simulink model "PV_MPPT"  (R2023a)
settings: Solver=VariableStepAuto  StartTime=0.0  StopTime=2  RelTol=1e-3
undefined symbols (not defined in the file): Ion, Lithium
libraries: spsSeriesRLCBranchLib x4, spsVariableResistorLib x2, spsVoltageMeasurementLib x2, spsBatteryLib x1, spsCurrentMeasurementLib x1, spsDiodeLib x1, spsIGBTLib x1, spsPVArrayLib x1, spspowerguiLib x1
settings Model: Creator=adity  LastModifiedBy=hp
settings RTWCC: GPUComputeCapability=5.0

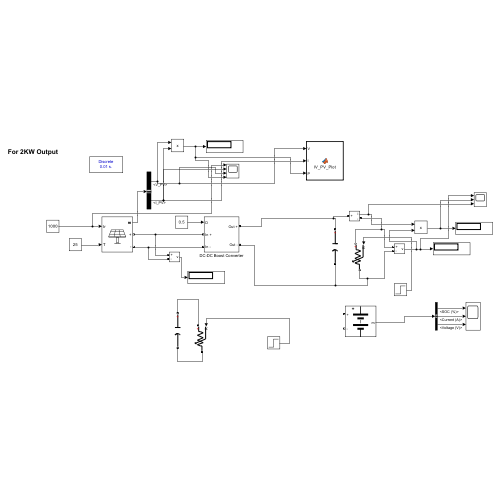
[thumbnail: Simulink's stored preview of the top-level diagram]
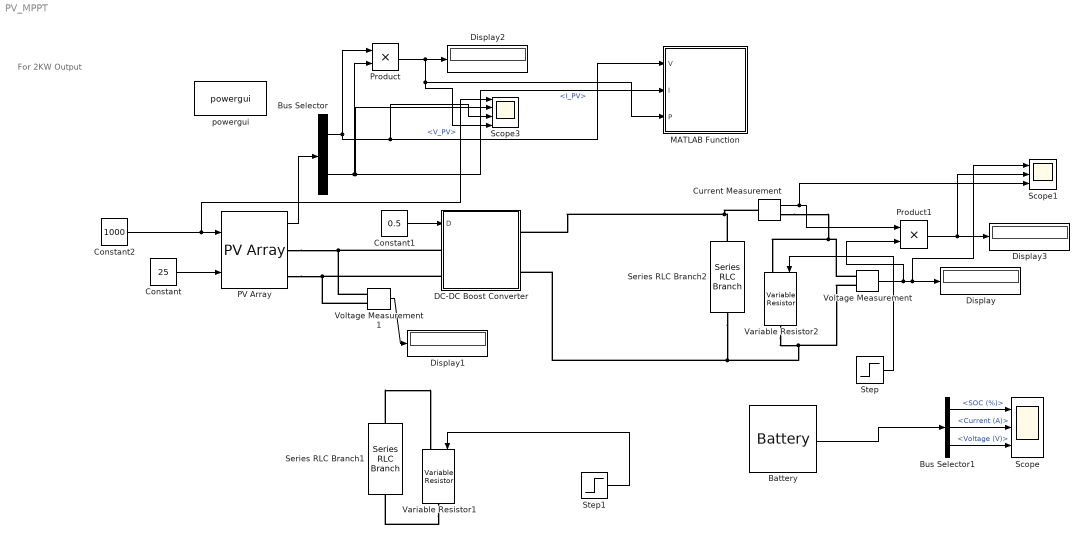
== system PV_MPPT ==
  note: For 2KW Output
  Battery : spsBatteryLib/Battery  BatType=Lithium-Ion  ShowTempParam=off  ThermalPreset=no  ShowAgeParam=off  NomV=7.2  NomQ=5.4  SOC=50  Batt_Tr=30  PresetModel=on  MaxQ=5.4  MinV=5.4  FullV=8.3807  Dis_rate=2.3478  R=0.013333  Normal_OP=4.8835  expZone="[7.7788      0.2653]"  current=[6.5 13 32.5]  Units=Time  Tci=20  NomT=20  T2=-30  MaxQ2=4.8  FullV2=7.1  Normal_OP2=5.655  expZone2="[6.58           1]"  Rca=0.6  ti=2000  Dp=0  Neq0=0  Tsim=1e6  Ta1=25  Qeol=5.4*0.9  Reol=0.013333*1.2  Char_age=[2.3478, 3]  Dis_age=[2.3478, 10]  N1=1500  N2=10500  N3=1000  N4=1400  Ta2=45  N5=950
  Bus Selector : BusSelector  OutputSignals=V_PV,I_PV
  Bus Selector1 : BusSelector  OutputSignals=SOC (%),Current (A),Voltage (V)
  Constant : Constant  Value=25
  Constant1 : Constant  Value=0.5
  Constant2 : Constant  Value=1000
  Current Measurement : spsCurrentMeasurementLib/Current Measurement  PhasorSimulation=off  OutputType=Complex  PSBequivalent=0
  DC-DC Boost Converter : Subsystem
  Display{,1..3} (4 alike) : Display
  MATLAB Function : MATLAB Function  TreatAsAtomicUnit=on
  PV Array : spsPVArrayLib/PV Array  Npar=1  Nser=10  PlotType=array @ 25 deg.C & specified irradiances  S_vec="[ 1000  800 600 400 200 ]"  Temp_C_vec="[ 45 25  ]"  ModuleName=Waaree Energies WU-200  PlotWhenSelected=off  Pm=200.2  Ncell=54  Voc=32  Isc=8.7  Vm=26  Im=7.7  beta_Voc_pc=-0.358  alpha_Isc_pc=0.052  beta_Voc=-0.11456  alpha_Isc=0.004524  IL=8.7534  I0=2.651e-10  nI=0.95585  Rsh=42.5034  Rs=0.26085  RobustModel=off  RobustCellTemperature=313.3991  BAL=on  Tc=1e-6  Tfilter=5e-5
  Product : Product
  Product1 : Product
  Scope : Scope  NumInputPorts=3
  Scope1 : Scope  NumInputPorts=3
  Scope3 : Scope  NumInputPorts=4
  Series RLC Branch1 : spsSeriesRLCBranchLib/Series RLC Branch  LConnTagsString=__new0  RConnTagsString=__new0  BranchType=C  Resistance=1  Inductance=1e-3  SetiL0=off  InitialCurrent=0  Capacitance=1200e-6  Setx0=off  InitialVoltage=0  Measurements=None
  Series RLC Branch2 : spsSeriesRLCBranchLib/Series RLC Branch  LConnTagsString=__new0  RConnTagsString=__new0  BranchType=C  Resistance=1  Inductance=1e-3  SetiL0=off  InitialCurrent=0  Capacitance=1200e-6  Setx0=off  InitialVoltage=0  Measurements=None
  Step : Step  Before=60  After=100  SampleTime=0
  Step1 : Step  Before=60  After=100  SampleTime=0
  Variable Resistor1 : spsVariableResistorLib/Variable Resistor  Rabsmin=1e-3
      settings: LibrarySourceBlock=sps_lib/Passives/Variable Resistor
  Variable Resistor2 : spsVariableResistorLib/Variable Resistor  Rabsmin=1e-3
      settings: LibrarySourceBlock=sps_lib/Passives/Variable Resistor
  Voltage Measurement : spsVoltageMeasurementLib/Voltage Measurement  PhasorSimulation=off  OutputType=Complex  PSBequivalent=0
  Voltage Measurement1 : spsVoltageMeasurementLib/Voltage Measurement  PhasorSimulation=off  OutputType=Complex  PSBequivalent=0
  powergui : spspowerguiLib/powergui  Priority=1  SimulationMode=Discrete  SampleTime=1e-2  frequency=60  Iterations=50  frequencyindice=0  Pbase=100e6  ErrMax=1e-4  UnitsV=kV  UnitsW=MW  buscounter=0  FunctionMessages=off  echomessages=off  EnableUseOfTLC=off  CurrentSourceSwitches=off  DisableSnubberDevices=off  DisableRonSwitches=off  DisableVfSwitches=off  DisplayEquations=off  AutomaticDiscreteSolvers=off  SolverType=Tustin/Backward Euler (TBE)  Interpol=off  ExternalGateDelay=off  methode=off  Ts=100  x0status=blocks  SPID=on  SwTol=0  HookPort=off  NonlinearTolerance=1e-4  nMaxIteration=100  ContinueOnMaxIteration=off  RestoreLinks=warning  ResistiveCurrentMeasurement=off  Frange=[0:2:500]  Ylog=off  Xlog=on  ShowGrid=off  save=off  variable=ZData  structure=0  ZoomFFT=off  StartTime=0.0  cycles=1  DisplayStyle=1  fundamental=60  FreqAxis=off  MaxFrequency=1000  frequencyindicesteady=1  RmsSteady=1  display=off
  wires:
  Constant/1 -> PV Array/2
  Constant2/1 -> Scope3/1, PV Array/1
  Voltage Measurement/1 -> Product1/2, Scope1/1, Display/1
  PV Array/1 -> Bus Selector/1
  Bus Selector/1 -> Product/1, MATLAB Function/1(V), Scope3/3  "<V_PV>"
  Bus Selector/2 -> MATLAB Function/2(I), Scope3/2, Product/2  "<I_PV>"
  Constant1/1 -> DC-DC Boost Converter/1(D)
  Voltage Measurement1/1 -> Display1/1
  Product/1 -> MATLAB Function/3(P), Scope3/4, Display2/1
  Current Measurement/1 -> Scope1/3, Product1/1
  Product1/1 -> Scope1/2, Display3/1
  Step/1 -> Variable Resistor2/1
  Step1/1 -> Variable Resistor1/1
  Battery/1 -> Bus Selector1/1
  Bus Selector1/1 -> Scope/1  "<SOC (%)>"
  Bus Selector1/2 -> Scope/2  "<Current (A)>"
  Bus Selector1/3 -> Scope/3  "<Voltage (V)>"
  connections:
  Voltage Measurement/LConn2 -- Variable Resistor2/RConn1 -- Series RLC Branch2/RConn1 -- DC-DC Boost Converter/RConn2
  Voltage Measurement/LConn1 -- Variable Resistor2/LConn1 -- Current Measurement/RConn1
  PV Array/RConn1 -- DC-DC Boost Converter/LConn1 -- Voltage Measurement1/LConn1
  Series RLC Branch2/LConn1 -- Current Measurement/LConn1 -- DC-DC Boost Converter/RConn1
  Voltage Measurement1/LConn2 -- DC-DC Boost Converter/LConn2 -- PV Array/RConn2
  Variable Resistor1/RConn1 -- Series RLC Branch1/RConn1
  Series RLC Branch1/LConn1 -- Variable Resistor1/LConn1

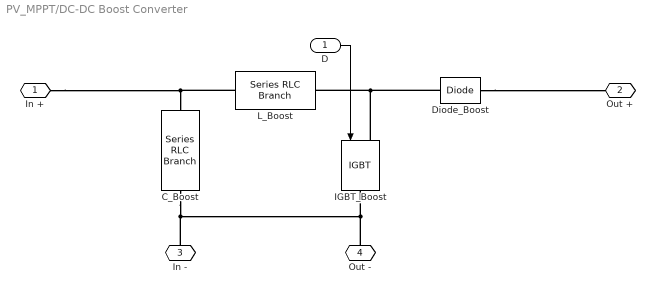
== system PV_MPPT/DC-DC Boost Converter ==
  D : Inport
  C_Boost : spsSeriesRLCBranchLib/Series RLC Branch  LConnTagsString=__new0  RConnTagsString=__new0  BranchType=C  Resistance=0.01  Inductance=1e-3  SetiL0=off  InitialCurrent=0  Capacitance=2200e-6  Setx0=off  InitialVoltage=0  Measurements=None
  Diode_Boost : spsDiodeLib/Diode  Ron=1e-4  Lon=0  Vf=0  IC=0  UseSnubber=off  Rs=inf  Cs=inf  Measurements=off
  IGBT_Boost : spsIGBTLib/IGBT  Ron=0.001  Lon=0  Vf=0  Tf=0  Tt=0  IC=0  Rs=1e5  Cs=inf  Measurements=off
  L_Boost : spsSeriesRLCBranchLib/Series RLC Branch  LConnTagsString=__new0  RConnTagsString=__new0  BranchType=RL  Resistance=0.05  Inductance=0.352e-3  SetiL0=off  InitialCurrent=0  Capacitance=1e-6  Setx0=off  InitialVoltage=0  Measurements=None
  In + : PMIOPort  Side=Left
  Out + : PMIOPort  Port=2  Side=Right
  In - : PMIOPort  Port=3  Side=Left
  Out - : PMIOPort  Port=4  Side=Right
  wires:
  D/1 -> IGBT_Boost/1
  connections:
  IGBT_Boost/LConn1 -- Diode_Boost/LConn1 -- L_Boost/RConn1
  Diode_Boost/RConn1 -- Out +/RConn1
  L_Boost/LConn1 -- In +/RConn1 -- C_Boost/LConn1
  C_Boost/RConn1 -- In -/RConn1 -- Out -/RConn1 -- IGBT_Boost/RConn1

== matlab function PV_MPPT/MATLAB Function ==
  data: V input; I input; P input
function IV_PV_Plot(V, I, P)
% This function plots I-V and P-V characteristics
% Inputs:
% V -> Voltage
% I -> Current
% P -> Power

persistent V_data I_data P_data

% Initialize arrays
if isempty(V_data)
    V_data = [];
    I_data = [];
    P_data = [];
end

% Store data
V_data = [V_data V];
I_data = [I_data I];
P_data = [P_data P];

% Plot I-V Characteristics
figure(1)
plot(V_data, I_data, 'b', 'LineWidth', 2)
xlabel('Voltage (V)')
ylabel('Current (A)')
title('I-V Characteristics of PV Array')
grid on

% Plot P-V Characteristics
figure(2)
plot(V_data, P_data, 'r', 'LineWidth', 2)
xlabel('Voltage (V)')
ylabel('Power (W)')
title('P-V Characteristics of PV Array')
grid on

end
